simulink model "chap13_7sim"  (Simulink 6.3)
settings: Solver=ode45  StartTime=0.0  StopTime=30  RelTol=1e-3
settings Model: LastModifiedBy=Administrator  ExtModeTrigMode=oneshot  ExtModeArmWhenConnect=off  StrictBusMsg=None
settings DataIOCC: LimitDataPoints=off  SignalLoggingName=sigsOut
settings OptimizationCC: BooleanDataType=off
settings DebuggingCC: SolverPrmCheckMsg=none
settings HardwareCC: TargetUnknown=on

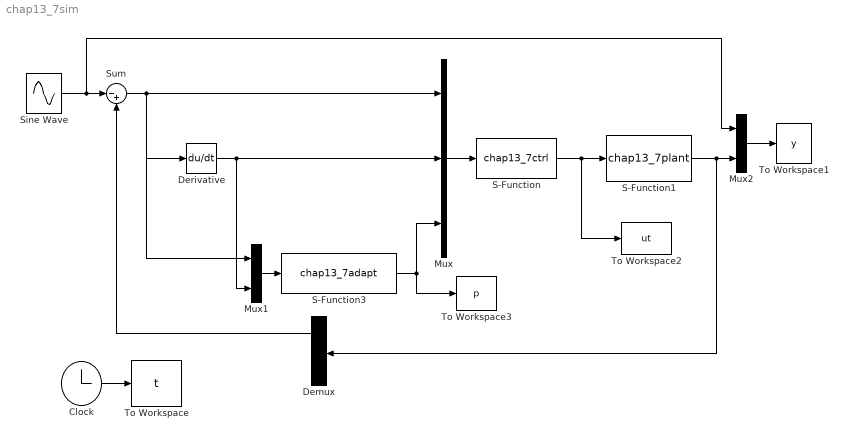
== system chap13_7sim ==
  Clock : Clock
  Demux : Demux  Orientation=left  Outputs=2
  Derivative : Derivative
  Mux : Mux  Inputs=3
  Mux1 : Mux  Inputs=2
  Mux2 : Mux  Inputs=2
  S-Function : S-Function  FunctionName=chap13_7ctrl
  S-Function1 : S-Function  FunctionName=chap13_7plant
  S-Function3 : S-Function  FunctionName=chap13_7adapt
  Sine Wave : Sin  SampleTime=0
  Sum : Sum  Inputs=|-+  SaturateOnIntegerOverflow=on
  To Workspace : ToWorkspace  VariableName=t  SampleTime=-1  SaveFormat=Array
  To Workspace1 : ToWorkspace  VariableName=y  SampleTime=-1  SaveFormat=Array
  To Workspace2 : ToWorkspace  VariableName=ut  SampleTime=-1  SaveFormat=Array
  To Workspace3 : ToWorkspace  VariableName=p  SampleTime=-1  SaveFormat=Array
  wires:
  S-Function/1 -> S-Function1/1, To Workspace2/1
  Clock/1 -> To Workspace/1
  S-Function1/1 -> Mux2/2, Demux/1
  Sine Wave/1 -> Sum/1, Mux2/1
  Mux/1 -> S-Function/1
  Sum/1 -> Mux/1, Derivative/1, Mux1/1
  Derivative/1 -> Mux/2, Mux1/2
  Mux1/1 -> S-Function3/1
  S-Function3/1 -> To Workspace3/1, Mux/3
  Mux2/1 -> To Workspace1/1
  Demux/1 -> Sum/2
